simulink model "half_car_active_model"  (R2018a)
settings: Solver=ode23t  StartTime=0.0  StopTime=50  MaxStep=0.001  RelTol=1e-3
values from neighbouring files (symbols this model uses):
  a = 0.675    [parameters.m]
  b = 0.6    [parameters.m]
  b1 = 3000    [parameters.m]
  b2 = 3000    [parameters.m]
  J = 48.96    [parameters.m]
  k1 = 190000    [parameters.m]
  k2 = 190000    [parameters.m]
  k3 = 16000    [parameters.m]
  k4 = 24000    [parameters.m]
  ms = 105    [parameters.m]
  mu_f = 25    [parameters.m]
  mu_r = 30    [parameters.m]
  td = L/(v*5/18)    (= 0.2655)    [parameters.m]
libraries: simulink x4, sdolib x1
settings Model: Creator=Saurabh Suman  LastModifiedBy=Saurabh Suman

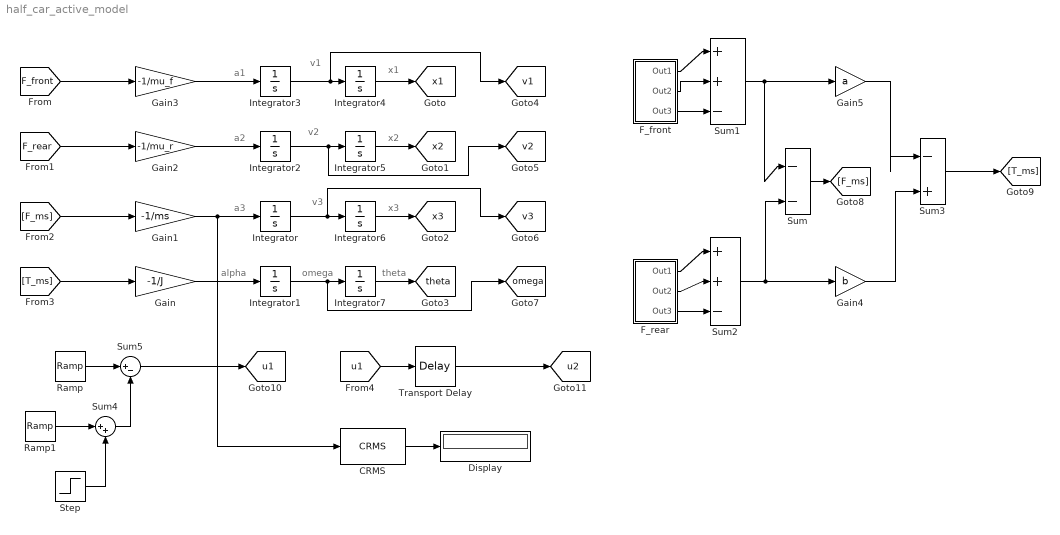
== system half_car_active_model ==
  note: omega
  note: v3
  note: theta
  note: v2
  note: a3
  note: v1
  note: a1
  note: x1
  note: a2
  note: x2
  note: x3
  note: alpha
  CRMS : sdolib/RMS Blocks/CRMS
      settings: SourceProductName=Simulink Design Optimization  SourceProductBaseCode=SO
  Display : Display
  F_front : Subsystem
  F_rear : Subsystem
  Gain : Gain  Gain=-1/J
  Gain1 : Gain  Gain=-1/ms
  Gain2 : Gain  Gain=-1/mu_r
  Gain3 : Gain  Gain=-1/mu_f
  Gain4 : Gain  Gain=b
  Gain5 : Gain  Gain=a
  Integrator{,1..7} (8 alike) : Integrator
  Ramp : simulink/Sources/Ramp  slope=0.125  start=1  InitialOutput=0
  Ramp1 : simulink/Sources/Ramp  slope=0.125  start=3  InitialOutput=0
  Step : Step  Time=3  After=0.25  SampleTime=0
  Sum : Sum  Inputs=|--
  Sum1 : Sum  Inputs=|++-
  Sum2 : Sum  Inputs=|++-
  Sum3 : Sum  Inputs=|-+
  Sum4 : Sum  Inputs=|++
  Sum5 : Sum  Inputs=|+-
  Transport Delay : TransportDelay  DelayTime=td
  tag scope: omega=global, theta=global, u1=global, u2=global, v1=global, v2=global, v3=global, x1=global, x2=global, x3=global
  wires:
  [F_ms] -> Gain1/1
  Integrator5/1 -> [x2]
  Integrator6/1 -> [x3]
  Gain5/1 -> Sum3/1
  Gain3/1 -> Integrator3/1
  Integrator2/1 -> [v2], Integrator5/1
  Integrator/1 -> [v3], Integrator6/1
  Sum2/1 -> Sum/2, Gain4/1
  Gain1/1 -> CRMS/1, Integrator/1
  F_front/1(Out1) -> Sum1/1
  Gain4/1 -> Sum3/2
  Integrator1/1 -> [omega], Integrator7/1
  F_rear/1(Out1) -> Sum2/1
  Integrator3/1 -> [v1], Integrator4/1
  F_rear/2(Out2) -> Sum2/2
  Gain/1 -> Integrator1/1
  F_front/2(Out2) -> Sum1/2
  Sum1/1 -> Sum/1, Gain5/1
  Integrator7/1 -> [theta]
  Gain2/1 -> Integrator2/1
  Integrator4/1 -> [x1]
  [T_ms] -> Gain/1
  [F_front] -> Gain3/1
  [F_rear] -> Gain2/1
  Sum/1 -> [F_ms]
  Sum3/1 -> [T_ms]
  F_rear/3(Out3) -> Sum2/3
  F_front/3(Out3) -> Sum1/3
  Sum5/1 -> [u1]
  Sum4/1 -> Sum5/2
  Ramp1/1 -> Sum4/1
  Ramp/1 -> Sum5/1
  Step/1 -> Sum4/2
  [u1] -> Transport Delay/1
  Transport Delay/1 -> [u2]
  CRMS/1 -> Display/1

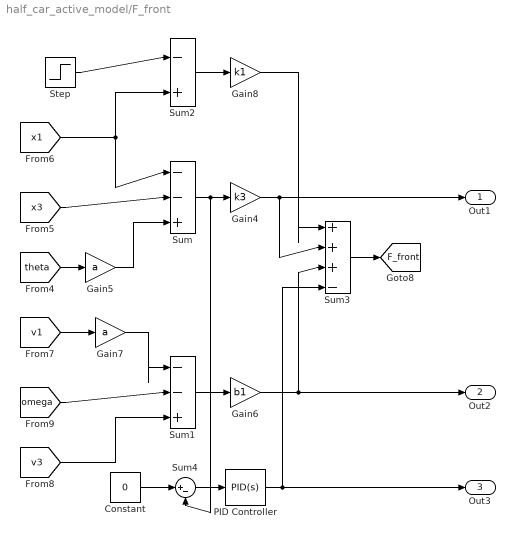
== system half_car_active_model/F_front ==
  Constant : Constant  Value=0
  Gain4 : Gain  Gain=k3
  Gain5 : Gain  Gain=a
  Gain6 : Gain  Gain=b1
  Gain7 : Gain  Gain=a
  Gain8 : Gain  Gain=k1
  PID Controller : simulink/Continuous/PID Controller  Controller=PID  TimeDomain=Continuous-time  SampleTime=-1  IntegratorMethod=Forward Euler  FilterMethod=Forward Euler  Form=Parallel  UseFilter=on  ControllerParametersSource=internal  P=1  I=1  D=0  N=100  InitialConditionSource=internal  InitialConditionForIntegrator=0  InitialConditionForFilter=0  ExternalReset=none  LimitOutput=off  UpperSaturationLimit=inf  LowerSaturationLimit=-inf  LinearizeAsGain=on  AntiWindupMode=none  Kb=1  TrackingMode=off  Kt=1  PParamMin=[]  PParamMax=[]  IParamMin=[]  IParamMax=[]  DParamMin=[]  DParamMax=[]  NParamMin=[]  NParamMax=[]  KbParamMin=[]  KbParamMax=[]  KtParamMin=[]  KtParamMax=[]  POutMin=[]  POutMax=[]  IOutMin=[]  IOutMax=[]  DOutMin=[]  DOutMax=[]  NOutMin=[]  NOutMax=[]  KbOutMin=[]  KbOutMax=[]  KtOutMin=[]  KtOutMax=[]  IntegratorOutMin=[]  IntegratorOutMax=[]  FilterOutMin=[]  FilterOutMax=[]  SumOutMin=[]  SumOutMax=[]  SumI1OutMin=[]  SumI1OutMax=[]  SumI2OutMin=[]  SumI2OutMax=[]  SumI3OutMin=[]  SumI3OutMax=[]  SumDOutMin=[]  SumDOutMax=[]  SaturationOutMin=[]  SaturationOutMax=[]  IntegratorContinuousStateAttributes=''  IntegratorStateMustResolveToSignalObject=off  IntegratorRTWStateStorageClass=Auto  FilterContinuousStateAttributes=''  FilterStateMustResolveToSignalObject=off  FilterRTWStateStorageClass=Auto  DifferentiatorICPrevScaledInput=0  DifferentiatorOutMin=[]  DifferentiatorOutMax=[]  FilterDiffOutCoefMin=[]  FilterDiffOutCoefMax=[]  SumDenOutMin=[]  SumDenOutMax=[]  SumNumOutMin=[]  SumNumOutMax=[]  ReciprocalOutMin=[]  ReciprocalOutMax=[]  DivideOutMin=[]  DivideOutMax=[]  TunerSelectOption=Transfer Function Based (PID Tuner App)
  Step : Step  SampleTime=0
  Sum : Sum  Inputs=|--+
  Sum1 : Sum  Inputs=|--+
  Sum2 : Sum  Inputs=|-+
  Sum3 : Sum  Inputs=|+++-
  Sum4 : Sum  Inputs=|+-
  Out1 : Outport
  Out2 : Outport  Port=2
  Out3 : Outport  Port=3
  tag scope: F_front=global
  wires:
  [v3] -> Sum1/3
  [theta] -> Gain5/1
  [v1] -> Gain7/1
  Step/1 -> Sum2/1
  Sum1/1 -> Gain6/1
  Gain5/1 -> Sum/3
  Gain4/1 -> Out1/1, Sum3/2
  Gain8/1 -> Sum3/1
  Gain6/1 -> Out2/1, Sum3/3
  Sum2/1 -> Gain8/1
  Gain7/1 -> Sum1/1
  [x1] -> Sum/1, Sum2/2
  [x3] -> Sum/2
  [omega] -> Sum1/2
  Sum3/1 -> [F_front]
  PID Controller/1 -> Sum3/4, Out3/1
  Constant/1 -> Sum4/1
  Sum/1 -> Sum4/2, Gain4/1
  Sum4/1 -> PID Controller/1

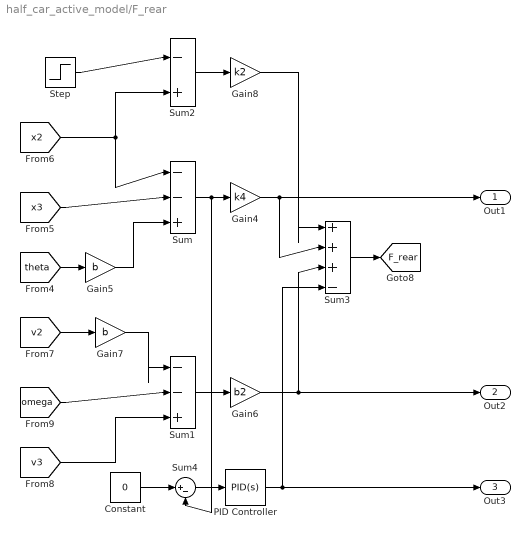
== system half_car_active_model/F_rear ==
  Constant : Constant  Value=0
  Gain4 : Gain  Gain=k4
  Gain5 : Gain  Gain=b
  Gain6 : Gain  Gain=b2
  Gain7 : Gain  Gain=b
  Gain8 : Gain  Gain=k2
  PID Controller : simulink/Continuous/PID Controller  Controller=PID  TimeDomain=Continuous-time  SampleTime=-1  IntegratorMethod=Forward Euler  FilterMethod=Forward Euler  Form=Parallel  UseFilter=on  ControllerParametersSource=internal  P=1  I=1  D=0  N=100  InitialConditionSource=internal  InitialConditionForIntegrator=0  InitialConditionForFilter=0  ExternalReset=none  LimitOutput=off  UpperSaturationLimit=inf  LowerSaturationLimit=-inf  LinearizeAsGain=on  AntiWindupMode=none  Kb=1  TrackingMode=off  Kt=1  PParamMin=[]  PParamMax=[]  IParamMin=[]  IParamMax=[]  DParamMin=[]  DParamMax=[]  NParamMin=[]  NParamMax=[]  KbParamMin=[]  KbParamMax=[]  KtParamMin=[]  KtParamMax=[]  POutMin=[]  POutMax=[]  IOutMin=[]  IOutMax=[]  DOutMin=[]  DOutMax=[]  NOutMin=[]  NOutMax=[]  KbOutMin=[]  KbOutMax=[]  KtOutMin=[]  KtOutMax=[]  IntegratorOutMin=[]  IntegratorOutMax=[]  FilterOutMin=[]  FilterOutMax=[]  SumOutMin=[]  SumOutMax=[]  SumI1OutMin=[]  SumI1OutMax=[]  SumI2OutMin=[]  SumI2OutMax=[]  SumI3OutMin=[]  SumI3OutMax=[]  SumDOutMin=[]  SumDOutMax=[]  SaturationOutMin=[]  SaturationOutMax=[]  IntegratorContinuousStateAttributes=''  IntegratorStateMustResolveToSignalObject=off  IntegratorRTWStateStorageClass=Auto  FilterContinuousStateAttributes=''  FilterStateMustResolveToSignalObject=off  FilterRTWStateStorageClass=Auto  DifferentiatorICPrevScaledInput=0  DifferentiatorOutMin=[]  DifferentiatorOutMax=[]  FilterDiffOutCoefMin=[]  FilterDiffOutCoefMax=[]  SumDenOutMin=[]  SumDenOutMax=[]  SumNumOutMin=[]  SumNumOutMax=[]  ReciprocalOutMin=[]  ReciprocalOutMax=[]  DivideOutMin=[]  DivideOutMax=[]  TunerSelectOption=Transfer Function Based (PID Tuner App)
  Step : Step  SampleTime=0
  Sum : Sum  Inputs=|--+
  Sum1 : Sum  Inputs=|--+
  Sum2 : Sum  Inputs=|-+
  Sum3 : Sum  Inputs=|+++-
  Sum4 : Sum  Inputs=|+-
  Out1 : Outport
  Out2 : Outport  Port=2
  Out3 : Outport  Port=3
  tag scope: F_rear=global
  wires:
  Gain6/1 -> Out2/1, Sum3/3
  Sum2/1 -> Gain8/1
  Sum3/1 -> [F_rear]
  [v2] -> Gain7/1
  [x3] -> Sum/2
  Gain4/1 -> Out1/1, Sum3/2
  [omega] -> Sum1/2
  [x2] -> Sum/1, Sum2/2
  Gain7/1 -> Sum1/1
  Step/1 -> Sum2/1
  [theta] -> Gain5/1
  Gain5/1 -> Sum/3
  Gain8/1 -> Sum3/1
  Sum/1 -> Sum4/2, Gain4/1
  [v3] -> Sum1/3
  Sum1/1 -> Gain6/1
  PID Controller/1 -> Sum3/4, Out3/1
  Constant/1 -> Sum4/1
  Sum4/1 -> PID Controller/1
